simulink model "cacc_manual"  (R2025a)
settings: Solver=VariableStepAuto  StartTime=0.0  StopTime=10.0  RelTol=1e-3
settings Model: Creator=matthewkeller  LastModifiedBy=matthewkeller

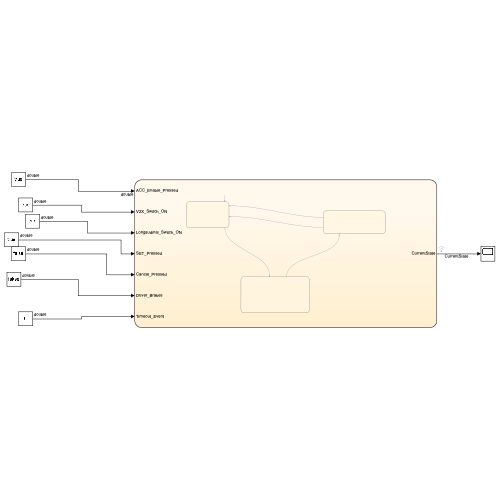
[thumbnail: Simulink's stored preview of the top-level diagram]
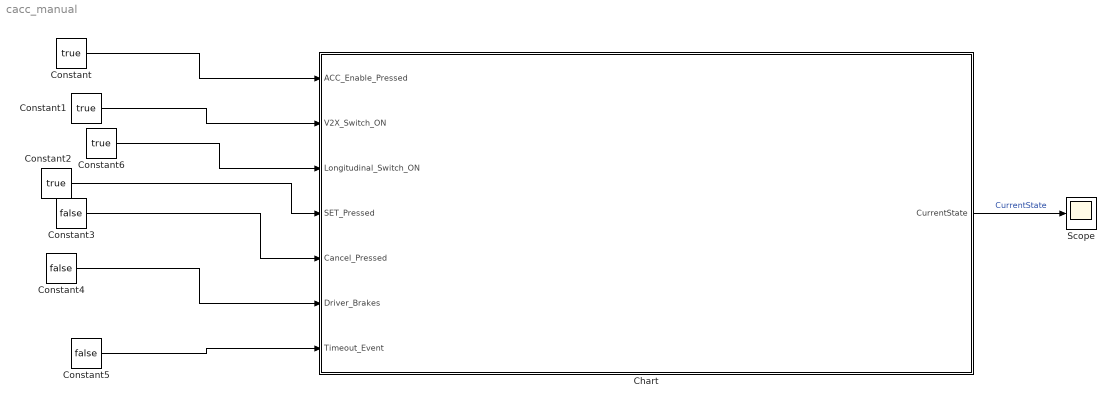
== system cacc_manual ==
  Chart : Stateflow chart  TreatAsAtomicUnit=on
  Constant{,1..2,6} (4 alike) : Constant  Value=true
  Constant3 : Constant  Value=false
  Constant4 : Constant  Value=false
  Constant5 : Constant  Value=false
  Scope : Scope
  wires:
  Chart/1(CurrentState) -> Scope/1  "CurrentState"
  Constant/1 -> Chart/1(ACC_Enable_Pressed)
  Constant5/1 -> Chart/7(Timeout_Event)
  Constant4/1 -> Chart/6(Driver_Brakes)
  Constant3/1 -> Chart/5(Cancel_Pressed)
  Constant2/1 -> Chart/4(SET_Pressed)
  Constant1/1 -> Chart/2(V2X_Switch_ON)
  Constant6/1 -> Chart/3(Longitudinal_Switch_ON)

== stateflow chart cacc_manual/Chart ==
  settings: executeAtInitialization=1
  state CACC_Deactivated
    entry:
    CurrentState = 0;
  state CACC_Active
    entry:
    CurrentState = 2;
  state CACC_Standby
    entry:
    CurrentState = 1;
  (default) -> CACC_Deactivated
  CACC_Active -> CACC_Deactivated [order 2] : [Timeout_Event]
  CACC_Active -> CACC_Deactivated [order 1] : [Cancel_Pressed || Driver_Brakes]
  CACC_Deactivated -> CACC_Standby : [ACC_Enable_Pressed && V2X_Switch_ON && Longitudinal_Switch_ON]
  CACC_Standby -> CACC_Active : [SET_Pressed]
  data: ACC_Enable_Pressed input boolean; V2X_Switch_ON input boolean; Longitudinal_Switch_ON input boolean; SET_Pressed input boolean; Cancel_Pressed input boolean; Driver_Brakes input boolean; Timeout_Event input boolean; CurrentState output int8
